simulink model "sgp4_unit_test"  (R2016b)
settings: Solver=FixedStepAuto  StartTime=0.0  StopTime=86400  RelTol=1e-3
values from neighbouring files (symbols this model uses):
  fsw_params = init_fsw_params()    [sgp4_stress_test_init.m]    (also in sgp4_test_init.m)
libraries: GPS_time_lib x1, sgp4_lib_fsw x1, time_coord_rotation_lib x1
settings Model: Creator=taylorreynolds  LastModifiedBy=taylorreynolds

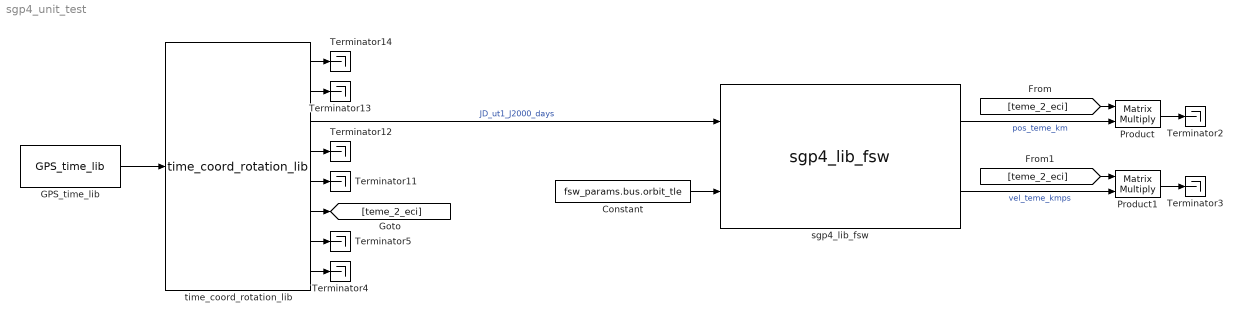
== system sgp4_unit_test ==
  Constant : Constant  Value=fsw_params.bus.orbit_tle
  GPS_time_lib : GPS_time_lib/GPS_time_lib
  Product : Product  Multiplication=Matrix(*)
  Product1 : Product  Multiplication=Matrix(*)
  Terminator{2..5,11..14} (8 alike) : Terminator
  sgp4_lib_fsw : sgp4_lib_fsw/sgp4_lib_fsw
  time_coord_rotation_lib : time_coord_rotation_lib/time_coord_rotation_lib
  wires:
  time_coord_rotation_lib/3 -> sgp4_lib_fsw/1  "JD_ut1_J2000_days"
  sgp4_lib_fsw/1 -> Product/2  "pos_teme_km"
  sgp4_lib_fsw/2 -> Product1/2  "vel_teme_kmps"
  Product/1 -> Terminator2/1
  Constant/1 -> sgp4_lib_fsw/2
  GPS_time_lib/1 -> time_coord_rotation_lib/1
  time_coord_rotation_lib/6 -> [teme_2_eci]
  [teme_2_eci] -> Product/1
  [teme_2_eci] -> Product1/1
  Product1/1 -> Terminator3/1
  time_coord_rotation_lib/8 -> Terminator4/1
  time_coord_rotation_lib/7 -> Terminator5/1
  time_coord_rotation_lib/5 -> Terminator11/1
  time_coord_rotation_lib/4 -> Terminator12/1
  time_coord_rotation_lib/2 -> Terminator13/1
  time_coord_rotation_lib/1 -> Terminator14/1
